simulink model "CSK_Std_PulseTrain_SlidingMode_Sect3"  (R2016b)
settings: Solver=ode45  StartTime=0.0  StopTime=400  RelTol=1e-10
values from neighbouring files (symbols this model uses):
  beta = 25.6    [RUN_021317.m]    (also in RUN_021417.m; RUN_022117.m)
  delay = 0    [RUN_022117.m]
  eta = 5    [RUN_110616.m]
  freq = message baud rate    [ErrChk.m]    (also in LoadText.m = Message Frequency; ProcessSync.m = expected bit frequency; ProcessSyncPeak.m = expected bit frequency; ProcessSyncPeak2.m = expected bit frequency)
  rho = 2    [RUN_021317.m]    (also in RUN_021417.m; RUN_022117.m)
  sig = 10    [RUN_021317.m]    (also in RUN_021417.m; RUN_022117.m)
  x0 = [.1,.2,.3]    [RUN_021317.m]    (also in RUN_021417.m; RUN_022117.m)
  z0 = x0    [RUN_021317.m]    (also in RUN_021417.m; RUN_022117.m)
settings Model: Creator=Dan  LastModifiedBy=Dan
settings DataIOCC: LimitDataPoints=on  SaveFormat=Array
settings OptimizationCC: BlockReduction=off  BooleanDataType=off  LifeSpan=inf
settings DebuggingCC: SaveWithParameterizedLinksMsg=none  UnderspecifiedInitializationDetection=Classic  MergeDetectMultiDrivingBlocksExec=none  SignalResolutionControl=TryResolveAllWithWarning  SFUnexpectedBacktrackingDiag=warning  SFNoUnconditionalDefaultTransitionDiag=warning  SFExecutionAtInitializationDiag=none
settings HardwareCC: ProdBitPerPointer=32  ProdBitPerSizeT=32  ProdBitPerPtrDiffT=32  ProdLargestAtomicFloat=None  ProdIntDivRoundTo=Undefined  ProdEndianess=Unspecified  ProdWordSize=32  ProdHWDeviceType=32-bit Generic  TargetUnknown=on
settings ModelReferenceCC: PropagateSignalLabelsOutOfModel=off
settings GRTTargetCC: TargetLangStandard=C89/C90 (ANSI)  GeneratePreprocessorConditionals=Disable all
settings ConfigComp: CovMetricSettings=dw  CovHtmlReporting=on  CovSaveCumulativeToWorkspaceVar=on  CovSaveSingleToWorkspaceVar=on  CovExternalEMLEnable=off  CovSFcnEnable=off

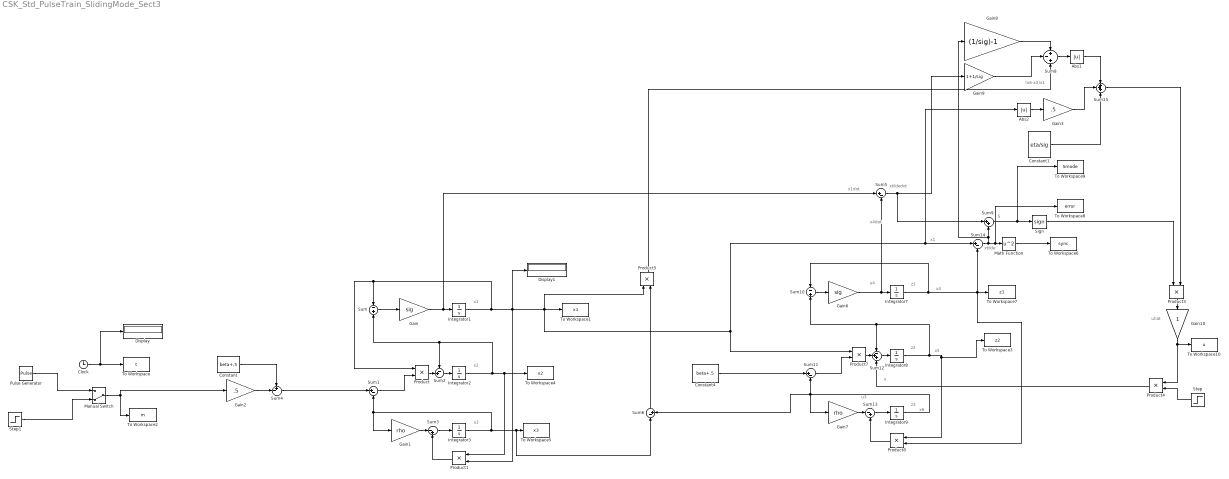
== system CSK_Std_PulseTrain_SlidingMode_Sect3 ==
  note: (x6-x3)x1
  note: uhat
  note: S
  note: x4
  note: x6
  note: x5
  note: xtildedot
  note: x4dot
  note: x1dot
  note: x1
  note: u
  note: xtilde
  note: u3
  note: u4
  note: x1
  note: x2
  note: x3
  note: z1
  note: z2
  note: z3
  Abs1 : Abs  ZeroCross=off
  Abs2 : Abs  ZeroCross=off
  Clock : Clock
  Constant : Constant  Value=beta+.5
  Constant1 : Constant  Value=eta/sig
  Constant4 : Constant  Value=beta+.5
  Display : Display
      settings: Decimation=5
  Display1 : Display
      settings: Decimation=5
  Gain : Gain  Gain=sig
  Gain1 : Gain  Gain=rho
  Gain10 : Gain
  Gain2 : Gain  Gain=.5
  Gain3 : Gain  Gain=.5
  Gain6 : Gain  Gain=sig
  Gain7 : Gain  Gain=rho
  Gain8 : Gain  Gain=(1/sig)-1
  Gain9 : Gain  Gain=1+1/sig
  Integrator1 : Integrator  InitialCondition=x0(1)
  Integrator2 : Integrator  InitialCondition=x0(2)
  Integrator3 : Integrator  InitialCondition=x0(3)
  Integrator7 : Integrator  InitialCondition=z0(1)
  Integrator8 : Integrator  InitialCondition=z0(2)
  Integrator9 : Integrator  InitialCondition=z0(3)
  Manual Switch : ManualSwitch  CurrentSetting=0
  Math Function : Math  Operator=square  SaturateOnIntegerOverflow=on
  Product{,1,3..5,7..8} (7 alike) : Product
  Pulse Generator : DiscretePulseGenerator  PulseType=Time based  Period=2/freq  PulseWidth=50  PhaseDelay=delay
  Sign : Signum  ZeroCross=off
  Step : Step  Time=0  SampleTime=0
  Step1 : Step  Time=delay  SampleTime=0
  Sum : Sum  Inputs=-|+
  Sum{1,5,11,14} (4 alike) : Sum  Inputs=|+-
  Sum10 : Sum  Inputs=-|+
  Sum12 : Sum  Inputs=-++
  Sum13 : Sum  Inputs=|-+
  Sum15 : Sum  Inputs=+++
  Sum2 : Sum  Inputs=-+|
  Sum3 : Sum  Inputs=|-+
  Sum4 : Sum  Inputs=+-|
  Sum6 : Sum  Inputs=|-+
  Sum8 : Sum  Inputs=+-+
  Sum9 : Sum  Inputs=|++
  To Workspace : ToWorkspace  VariableName=t  SampleTime=-1
  To Workspace1 : ToWorkspace  VariableName=x1  SampleTime=-1
  To Workspace10 : ToWorkspace  VariableName=u  SampleTime=-1
  To Workspace2 : ToWorkspace  VariableName=m  SampleTime=-1
  To Workspace3 : ToWorkspace  VariableName=z2  SampleTime=-1
  To Workspace4 : ToWorkspace  VariableName=x2  SampleTime=-1
  To Workspace5 : ToWorkspace  VariableName=x3  SampleTime=-1
  To Workspace6 : ToWorkspace  VariableName=sync  SampleTime=-1
  To Workspace7 : ToWorkspace  VariableName=z1  SampleTime=-1
  To Workspace8 : ToWorkspace  VariableName=error  SampleTime=-1
  To Workspace9 : ToWorkspace  VariableName=Smode  SampleTime=-1
  wires:
  Gain/1 -> Sum5/1, Integrator1/1
  Sum/1 -> Gain/1
  Sum1/1 -> Product/2
  Integrator3/1 -> Sum6/1, To Workspace5/1, Gain1/1, Sum1/2
  Sum3/1 -> Integrator3/1
  Product1/1 -> Sum3/2
  Integrator2/1 -> To Workspace4/1, Product1/1, Sum2/1, Sum/2
  Gain1/1 -> Sum3/1
  Gain2/1 -> Sum4/2
  Constant/1 -> Sum4/1
  Sum4/1 -> Sum1/1
  Clock/1 -> Display/1, To Workspace/1
  Product/1 -> Sum2/2
  Sum2/1 -> Integrator2/1
  Sum10/1 -> Gain6/1
  Sum11/1 -> Product7/2
  Sum13/1 -> Integrator9/1
  Product7/1 -> Sum12/2
  Sum12/1 -> Integrator8/1
  Integrator7/1 -> Product8/2, To Workspace7/1, Sum14/2, Sum10/1
  Sum14/1 -> Gain8/1, Sum9/2, To Workspace8/1, Math Function/1
  Integrator1/1 -> Sum/1, Product/1, Product1/2, Display1/1, Product5/1, Product7/1, Abs2/1, Sum14/1, To Workspace1/1
  Math Function/1 -> To Workspace6/1
  Gain6/1 -> Sum5/2, Integrator7/1
  Integrator8/1 -> To Workspace3/1, Product8/1, Sum12/1, Sum10/2
  Integrator9/1 -> Sum6/2, Sum11/2, Gain7/1
  Gain7/1 -> Sum13/1
  Product8/1 -> Sum13/2
  Constant4/1 -> Sum11/1
  Sum5/1 -> Gain9/1, Sum9/1
  Sum9/1 -> Sign/1, To Workspace9/1
  Sum15/1 -> Product3/2
  Sign/1 -> Product3/1
  Step/1 -> Product4/2
  Product4/1 -> Sum12/3
  Product3/1 -> Gain10/1
  Pulse Generator/1 -> Manual Switch/1
  Manual Switch/1 -> Gain2/1, To Workspace2/1
  Step1/1 -> Manual Switch/2
  Gain10/1 -> To Workspace10/1, Product4/1
  Sum8/1 -> Abs1/1
  Gain8/1 -> Sum8/1
  Gain9/1 -> Sum8/2
  Product5/1 -> Sum8/3
  Constant1/1 -> Sum15/3
  Sum6/1 -> Product5/2
  Abs1/1 -> Sum15/1
  Gain3/1 -> Sum15/2
  Abs2/1 -> Gain3/1
